simulink subsystem "VCM_main_Acc2"  (R2021b)
settings: Solver=VariableStepAuto  StartTime=0.0  StopTime=10.0  RelTol=1e-3
undefined symbols (not defined in the file): df, dr, g, gear_f, gear_r, Iwf, Iwr, l, lf, M, Rwf, Rwr
libraries: simulink x43, dspstat3 x2, dspswit3 x1
(part 1 of 3)
settings Model: Creator=tsuyoshi  LastModifiedBy=FEM

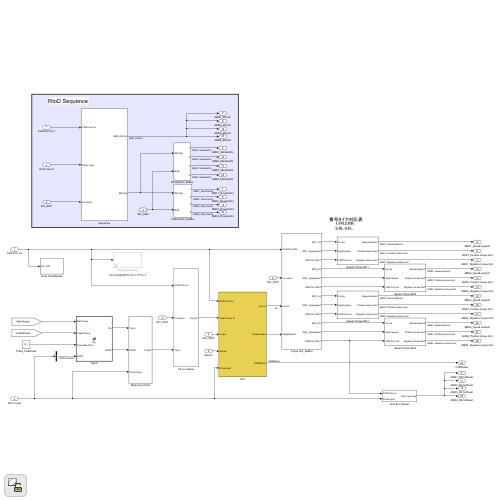
[thumbnail: Simulink's stored preview of the top-level diagram]
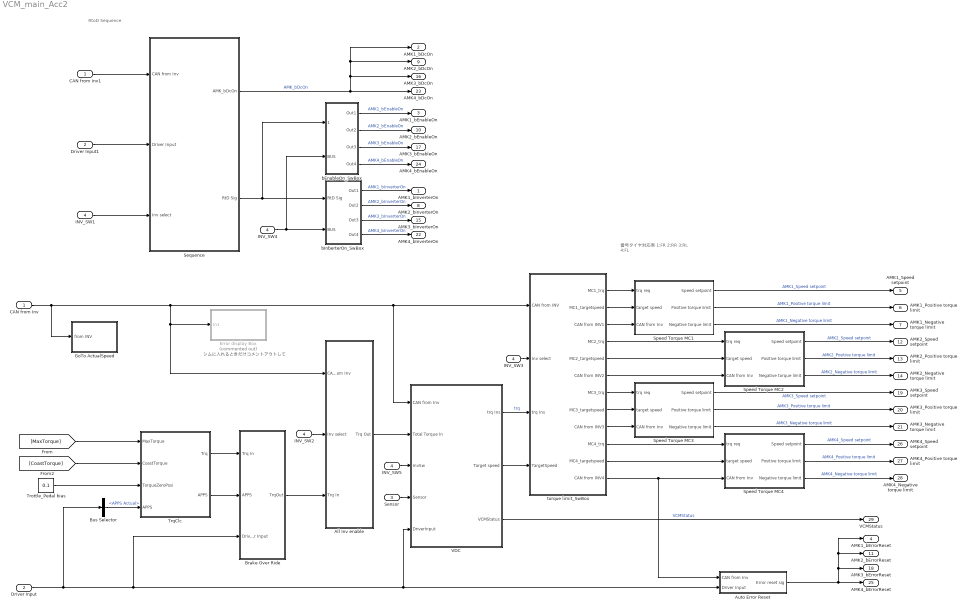
== system VCM_main_Acc2 ==
  note: シムに入れるときだけコメントアウトして
  note: RtoD Sequence
  note: 番号タイヤ対応表
      | 1:FR 2:RR
      | 3:RL 4:FL
  CAN from Inv : Inport
  Driver Input : Inport  Port=2
  Sensor : Inport  Port=3
  INV_SW1 : Inport  Port=4
  All Inv enable : Subsystem
  Auto Error Reset : Subsystem
  Brake Over Ride : Subsystem
  Bus Selector : BusSelector  OutputSignals=APPS Actual
  CAN from Inv1 : InportShadow
  Driver Input1 : InportShadow  Port=2
  Error display Box : Subsystem  Commented=on
  GoTo ActualSpeed : Subsystem
  INV_SW{2..5} (4 alike) : InportShadow  Port=4
  Sequence : Subsystem
  Speed Torque MC1 : Subsystem
  Speed Torque MC2 : Subsystem
  Speed Torque MC3 : Subsystem
  Speed Torque MC4 : Subsystem
  Trottle_Pedal bias : Constant  Value=0.1
  TrqClc : MATLAB Function  TreatAsAtomicUnit=on
  VDC : Subsystem
  bEnableOn_SwBox : Subsystem
  bInberterOn_SwBox : Subsystem
  torque limit_SwBox : Subsystem
  AMK1_bInverterOn : Outport  VectorParamsAs1DForOutWhenUnconnected=off
  AMK1_bDcOn : Outport  Port=2  VectorParamsAs1DForOutWhenUnconnected=off
  AMK1_bEnableOn : Outport  Port=3  VectorParamsAs1DForOutWhenUnconnected=off
  AMK1_bErrorReset : Outport  Port=4  VectorParamsAs1DForOutWhenUnconnected=off
  AMK1_Speed setpoint : Outport  Port=5  VectorParamsAs1DForOutWhenUnconnected=off
  AMK1_Positive torque limit : Outport  Port=6  VectorParamsAs1DForOutWhenUnconnected=off
  AMK1_Negative torque limit : Outport  Port=7  VectorParamsAs1DForOutWhenUnconnected=off
  AMK2_bInverterOn : Outport  Port=8  VectorParamsAs1DForOutWhenUnconnected=off
  AMK2_bDcOn : Outport  Port=9  VectorParamsAs1DForOutWhenUnconnected=off
  AMK2_bEnableOn : Outport  Port=10  VectorParamsAs1DForOutWhenUnconnected=off
  AMK2_bErrorReset : Outport  Port=11  VectorParamsAs1DForOutWhenUnconnected=off
  AMK2_Speed setpoint : Outport  Port=12  VectorParamsAs1DForOutWhenUnconnected=off
  AMK2_Positive torque limit : Outport  Port=13  VectorParamsAs1DForOutWhenUnconnected=off
  AMK2_Negative torque limit : Outport  Port=14  VectorParamsAs1DForOutWhenUnconnected=off
  AMK3_bInverterOn : Outport  Port=15  VectorParamsAs1DForOutWhenUnconnected=off
  AMK3_bDcOn : Outport  Port=16  VectorParamsAs1DForOutWhenUnconnected=off
  AMK3_bEnableOn : Outport  Port=17  VectorParamsAs1DForOutWhenUnconnected=off
  AMK3_bErrorReset : Outport  Port=18  VectorParamsAs1DForOutWhenUnconnected=off
  AMK3_Speed setpoint : Outport  Port=19  VectorParamsAs1DForOutWhenUnconnected=off
  AMK3_Positive torque limit : Outport  Port=20  VectorParamsAs1DForOutWhenUnconnected=off
  AMK3_Negative torque limit : Outport  Port=21  VectorParamsAs1DForOutWhenUnconnected=off
  AMK4_bInverterOn : Outport  Port=22  VectorParamsAs1DForOutWhenUnconnected=off
  AMK4_bDcOn : Outport  Port=23  VectorParamsAs1DForOutWhenUnconnected=off
  AMK4_bEnableOn : Outport  Port=24  VectorParamsAs1DForOutWhenUnconnected=off
  AMK4_bErrorReset : Outport  Port=25  VectorParamsAs1DForOutWhenUnconnected=off
  AMK4_Speed setpoint : Outport  Port=26  VectorParamsAs1DForOutWhenUnconnected=off
  AMK4_Positive torque limit : Outport  Port=27  VectorParamsAs1DForOutWhenUnconnected=off
  AMK4_Negative torque limit : Outport  Port=28  VectorParamsAs1DForOutWhenUnconnected=off
  VCMStatus : Outport  Port=29  VectorParamsAs1DForOutWhenUnconnected=off
  wires:
  Sequence/1(AMK_bDcOn) -> AMK4_bDcOn/1, AMK3_bDcOn/1, AMK2_bDcOn/1, AMK1_bDcOn/1  "AMK_bDcOn"
  Trottle_Pedal bias/1 -> TrqClc/3(TorqueZeroPosi)
  bInberterOn_SwBox/1(Out1) -> AMK1_bInverterOn/1  "AMK1_bInverterOn"
  bInberterOn_SwBox/2(Out2) -> AMK2_bInverterOn/1  "AMK2_bInverterOn"
  bInberterOn_SwBox/3(Out3) -> AMK3_bInverterOn/1  "AMK3_bInverterOn"
  bInberterOn_SwBox/4(Out4) -> AMK4_bInverterOn/1  "AMK4_bInverterOn"
  INV_SW1/1 -> Sequence/3(Inv select)
  bEnableOn_SwBox/1(Out1) -> AMK1_bEnableOn/1  "AMK1_bEnableOn"
  bEnableOn_SwBox/2(Out2) -> AMK2_bEnableOn/1  "AMK2_bEnableOn"
  bEnableOn_SwBox/3(Out3) -> AMK3_bEnableOn/1  "AMK3_bEnableOn"
  bEnableOn_SwBox/4(Out4) -> AMK4_bEnableOn/1  "AMK4_bEnableOn"
  Sequence/2(RtD Sig) -> bEnableOn_SwBox/1(RtD Sig), bInberterOn_SwBox/1(RtD Sig)
  VDC/1(trq Ins) -> torque limit_SwBox/3(trq Ins)  "trq"
  CAN from Inv/1 -> GoTo ActualSpeed/1(from INV), torque limit_SwBox/1(CAN from INV), VDC/1(CAN from Inv), All Inv enable/1(CAN from Inv), Error display Box/1(In1)
  TrqClc/1(Trq) -> Brake Over Ride/1(Trq In)
  Brake Over Ride/1(TrqOut) -> All Inv enable/3(Trq In)
  All Inv enable/1(Trq Out) -> VDC/2(Total Torque In)
  torque limit_SwBox/1(MC1_trq) -> Speed Torque MC1/1(trq req)
  Speed Torque MC1/1(Speed setpoint) -> AMK1_Speed setpoint/1  "AMK1_Speed setpoint"
  Speed Torque MC1/2(Positive torque limit) -> AMK1_Positive torque limit/1  "AMK1_Positive torque limit"
  Speed Torque MC1/3(Negative torque limit) -> AMK1_Negative torque limit/1  "AMK1_Negative torque limit"
  Speed Torque MC2/1(Speed setpoint) -> AMK2_Speed setpoint/1  "AMK2_Speed setpoint"
  Speed Torque MC2/2(Positive torque limit) -> AMK2_Positive torque limit/1  "AMK2_Positive torque limit"
  Speed Torque MC2/3(Negative torque limit) -> AMK2_Negative torque limit/1  "AMK2_Negative torque limit"
  torque limit_SwBox/4(MC2_trq) -> Speed Torque MC2/1(trq req)
  Speed Torque MC3/1(Speed setpoint) -> AMK3_Speed setpoint/1  "AMK3_Speed setpoint"
  Speed Torque MC3/2(Positive torque limit) -> AMK3_Positive torque limit/1  "AMK3_Positive torque limit"
  Speed Torque MC3/3(Negative torque limit) -> AMK3_Negative torque limit/1  "AMK3_Negative torque limit"
  Speed Torque MC4/1(Speed setpoint) -> AMK4_Speed setpoint/1  "AMK4_Speed setpoint"
  Speed Torque MC4/2(Positive torque limit) -> AMK4_Positive torque limit/1  "AMK4_Positive torque limit"
  Speed Torque MC4/3(Negative torque limit) -> AMK4_Negative torque limit/1  "AMK4_Negative torque limit"
  torque limit_SwBox/7(MC3_trq) -> Speed Torque MC3/1(trq req)
  torque limit_SwBox/10(MC4_trq) -> Speed Torque MC4/1(trq req)
  Auto Error Reset/1(Error reset sig) -> AMK4_bErrorReset/1, AMK3_bErrorReset/1, AMK1_bErrorReset/1, AMK2_bErrorReset/1
  Sensor/1 -> VDC/4(Sensor)
  torque limit_SwBox/2(MC1_targetspeed) -> Speed Torque MC1/2(target speed)
  torque limit_SwBox/8(MC3_targetspeed) -> Speed Torque MC3/2(target speed)
  torque limit_SwBox/5(MC2_targetspeed) -> Speed Torque MC2/2(target speed)
  torque limit_SwBox/11(MC4_targetspeed) -> Speed Torque MC4/2(target speed)
  VDC/3(VCMStatus) -> VCMStatus/1  "VCMStatus"
  VDC/2(Target speed) -> torque limit_SwBox/4(TargetSpeed)
  INV_SW2/1 -> All Inv enable/2(Inv select)
  INV_SW3/1 -> torque limit_SwBox/2(Inv select)
  INV_SW4/1 -> bInberterOn_SwBox/2(BUS), bEnableOn_SwBox/2(BUS)
  torque limit_SwBox/3(CAN from INV1) -> Speed Torque MC1/3(CAN from Inv)
  torque limit_SwBox/6(CAN from INV2) -> Speed Torque MC2/3(CAN from Inv)
  torque limit_SwBox/9(CAN from INV3) -> Speed Torque MC3/3(CAN from Inv)
  torque limit_SwBox/12(CAN from INV4) -> Auto Error Reset/1(CAN from Inv), Speed Torque MC4/3(CAN from Inv)
  [MaxTorque] -> TrqClc/1(MaxTorque)
  Driver Input1/1 -> Sequence/2(Driver Input)
  CAN from Inv1/1 -> Sequence/1(CAN from Inv)
  [CoastTorque] -> TrqClc/2(CoastTorque)
  Bus Selector/1 -> TrqClc/4("APPS ")  "<APPS Actual>"
  TrqClc/2(APPS) -> Brake Over Ride/2(APPS)
  INV_SW5/1 -> VDC/3(InvSw)
  Driver Input/1 -> Brake Over Ride/3(Driver Input), VDC/5(DriverInput), Auto Error Reset/2(Driver Input), Bus Selector/1

== system VCM_main_Acc2/All Inv enable ==
  note: インバータがQuitInverterOnになる前にトルク指令値を送ってはいけない
  CAN from Inv : Inport
  Inv select : Inport  Port=2
  Trq In : Inport  Port=3
  All Inv enable : Subsystem
  Constant : Constant  Value=0
  Switch : Switch  Criteria=u2 ~= 0
  Trq Out : Outport  VectorParamsAs1DForOutWhenUnconnected=off
  wires:
  CAN from Inv/1 -> All Inv enable/1(CAN from Inv)
  Inv select/1 -> All Inv enable/2(Inv select)
  Trq In/1 -> Switch/1
  Switch/1 -> Trq Out/1
  All Inv enable/1(Out1) -> Switch/2
  Constant/1 -> Switch/3

== system VCM_main_Acc2/Auto Error Reset ==
  note: AutoErrorResetにしたいときは
      | これを下につなげる
  CAN from Inv : Inport
  Driver Input : Inport  Port=2
  Bus Selector : BusSelector  OutputSignals=ErrorResetSW
  Bus Selector1 : BusSelector  OutputSignals=MC_11.MC1_bError,MC_21.MC2_bError,MC_31.MC3_bError,MC_41.MC4_bError
  Counter : dspswit3/Counter  Direction=Up  CountEvent=Rising edge  CounterSize=User defined  MaxCount=5  InitialCount=0  Output=Hit  HitValue=5  ResetInput=on  SamplesPerFrame=1  Ts=1  CntDtype=double  HitDtype=Logical
  Data Type Conversion : DataTypeConversion  OutMin=[0]  OutMax=[1]  OutDataTypeStr=double
  Delay : Delay  DelayLength=1  InitialCondition=0
  Logical Operator : Logic  Operator=OR  AllPortsSameDT=off  OutDataTypeStr=boolean
  Logical Operator1 : Logic  Operator=OR  Inputs=4  AllPortsSameDT=off  OutDataTypeStr=boolean
  Logical Operator2 : Logic  AllPortsSameDT=off  OutDataTypeStr=boolean
  Logical Operator3 : Logic  Operator=NOT  AllPortsSameDT=off  OutDataTypeStr=boolean
  Logical Operator4 : Logic  Operator=OR  AllPortsSameDT=off  OutDataTypeStr=boolean
  Pulse Generator : DiscretePulseGenerator  PulseType=Time based  Period=60  PulseWidth=5
  Terminator : Terminator
  Error reset sig : Outport  VectorParamsAs1DForOutWhenUnconnected=off
  wires:
  Logical Operator/1 -> Terminator/1
  Data Type Conversion/1 -> Error reset sig/1  "AMK_bErrorReset"
  Bus Selector1/4 -> Logical Operator1/4  "<MC4_bError>"
  Bus Selector1/3 -> Logical Operator1/3  "<MC3_bError>"
  Bus Selector1/1 -> Logical Operator1/1  "<MC1_bError>"
  Bus Selector1/2 -> Logical Operator1/2  "<MC2_bError>"
  Pulse Generator/1 -> Counter/2
  Delay/1 -> Logical Operator4/2
  Counter/1 -> Logical Operator4/1
  Logical Operator4/1 -> Delay/1, Logical Operator3/1
  Logical Operator2/1 -> Logical Operator/1
  Logical Operator3/1 -> Logical Operator2/2
  Logical Operator1/1 -> Counter/1, Logical Operator2/1
  CAN from Inv/1 -> Bus Selector1/1
  Bus Selector/1 -> Logical Operator/2, Data Type Conversion/1  "<ErrorResetSW>"
  Driver Input/1 -> Bus Selector/1

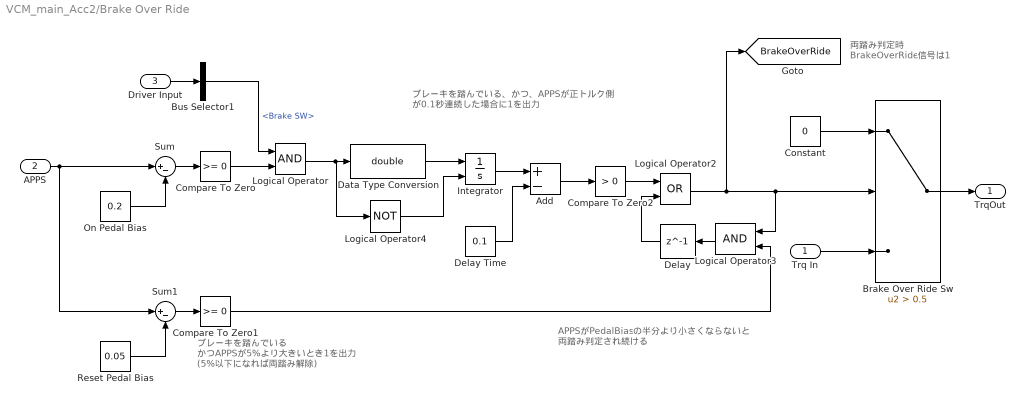
== system VCM_main_Acc2/Brake Over Ride ==
  note: APPSがPedalBiasの半分より小さくならないと
      | 両踏み判定され続ける
  note: ブレーキを踏んでいる
      | かつAPPSが5%より大きいとき1を出力
      | (5%以下になれば両踏み解除)
  note: 両踏み判定時
      | BrakeOverRide信号は1
  note: ブレーキを踏んでいる、かつ、APPSが正トルク側
      | が0.1秒連続した場合に1を出力
  Trq In : Inport
  APPS : Inport  Port=2
  Driver Input : Inport  Port=3
  Add : Sum  Inputs=+-
  Brake Over Ride Sw : Switch  Criteria=u2 > Threshold  Threshold=0.5
  Bus Selector1 : BusSelector  OutputSignals=Brake SW
  Compare To Zero : simulink/Logic and Bit Operations/Compare To Zero  relop=>=  OutDataTypeStr=boolean
  Compare To Zero1 : simulink/Logic and Bit Operations/Compare To Zero  relop=>=  OutDataTypeStr=boolean
  Compare To Zero2 : simulink/Logic and Bit Operations/Compare To Zero  relop=>  OutDataTypeStr=boolean
  Constant : Constant  Value=0
  Data Type Conversion : DataTypeConversion  OutDataTypeStr=double
  Delay : Delay  DelayLength=1  InitialCondition=0
  Delay Time : Constant  Value=0.1
  Integrator : Integrator  ExternalReset=rising
  Logical Operator : Logic  AllPortsSameDT=off  OutDataTypeStr=boolean
  Logical Operator2 : Logic  Operator=OR  AllPortsSameDT=off  OutDataTypeStr=boolean
  Logical Operator3 : Logic  AllPortsSameDT=off  OutDataTypeStr=boolean
  Logical Operator4 : Logic  Operator=NOT  AllPortsSameDT=off  OutDataTypeStr=boolean
  On Pedal Bias : Constant  Value=0.2
  Reset Pedal Bias : Constant  Value=0.05
  Sum : Sum  Inputs=|+-
  Sum1 : Sum  Inputs=|+-
  TrqOut : Outport  VectorParamsAs1DForOutWhenUnconnected=off
  tag scope: BrakeOverRide=global
  wires:
  Constant/1 -> Brake Over Ride Sw/1
  Brake Over Ride Sw/1 -> TrqOut/1
  Delay Time/1 -> Add/2
  Logical Operator/1 -> Data Type Conversion/1, Logical Operator4/1
  Integrator/1 -> Add/1
  Reset Pedal Bias/1 -> Sum1/2
  Sum/1 -> Compare To Zero/1
  Driver Input/1 -> Bus Selector1/1
  Logical Operator4/1 -> Integrator/2
  Logical Operator3/1 -> Delay/1
  Trq In/1 -> Brake Over Ride Sw/3
  Bus Selector1/1 -> Logical Operator/1  "<Brake SW>"
  APPS/1 -> Sum1/1, Sum/1
  Delay/1 -> Logical Operator2/2
  Data Type Conversion/1 -> Integrator/1
  Sum1/1 -> Compare To Zero1/1
  Compare To Zero2/1 -> Logical Operator2/1
  Compare To Zero/1 -> Logical Operator/2
  On Pedal Bias/1 -> Sum/2
  Logical Operator2/1 -> [BrakeOverRide], Logical Operator3/1, Brake Over Ride Sw/2
  Compare To Zero1/1 -> Logical Operator3/2
  Add/1 -> Compare To Zero2/1

== system VCM_main_Acc2/Error display Box ==
  note: 過去のエラーメッセージを見れるようにするためにある
  In1 : Inport
  All system ready : Logic  Inputs=4  AllPortsSameDT=off  OutDataTypeStr=boolean
  Bus Selector : BusSelector  OutputSignals=MC_11.MC1_bSystemReady,MC_21.MC2_bSystemReady,MC_31.MC3_bSystemReady,MC_41.MC4_bSystemReady
  Display : Display
  Error Info : Subsystem
  Error Info Display{,1..3} (4 alike) : Display
  Error Info1 : Subsystem
  Error Info2 : Subsystem
  Error Info3 : Subsystem
  wires:
  All system ready/1 -> Display/1
  Bus Selector/4 -> All system ready/4  "<MC4_bSystemReady>"
  Bus Selector/3 -> All system ready/3  "<MC3_bSystemReady>"
  Bus Selector/2 -> All system ready/2  "<MC2_bSystemReady>"
  Bus Selector/1 -> All system ready/1  "<MC1_bSystemReady>"
  Error Info/2(Out2) -> Error Info3/2(In2), Error Info2/2(In2), Error Info1/2(In2)
  Error Info3/1(Out1) -> Error Info Display3/1
  Error Info2/1(Out1) -> Error Info Display2/1
  Error Info1/1(Out1) -> Error Info Display1/1
  In1/1 -> Error Info/1(In1), Error Info1/1(In1), Error Info2/1(In1), Error Info3/1(In1), Bus Selector/1
  Error Info/1(Out1) -> Error Info Display/1

== system VCM_main_Acc2/GoTo ActualSpeed ==
  note: 番号タイヤ対応表
      | 1:FR 2:RR
      | 3:RL 4:FL
  from INV : Inport
  Bus Selector : BusSelector  OutputSignals=MC_11.MC1_Actual speed value in 1/rpm,MC_21.MC2_Actual speed value in 1/rpm,MC_31.MC3_Actual speed value in 1/rpm,MC_41.MC4_Actual speed value in 1/rpm
  tag scope: FL_ActualSpeed=global, FR_ActualSpeed=global, RL_ActualSpeed=global, RR_ActualSpeed=global
  wires:
  Bus Selector/4 -> [FL_ActualSpeed]  "<MC4_Actual speed value in 1/rpm>"
  Bus Selector/3 -> [RL_ActualSpeed]  "<MC3_Actual speed value in 1/rpm>"
  Bus Selector/2 -> [RR_ActualSpeed]  "<MC2_Actual speed value in 1/rpm>"
  Bus Selector/1 -> [FR_ActualSpeed]  "<MC1_Actual speed value in 1/rpm>"
  from INV/1 -> Bus Selector/1

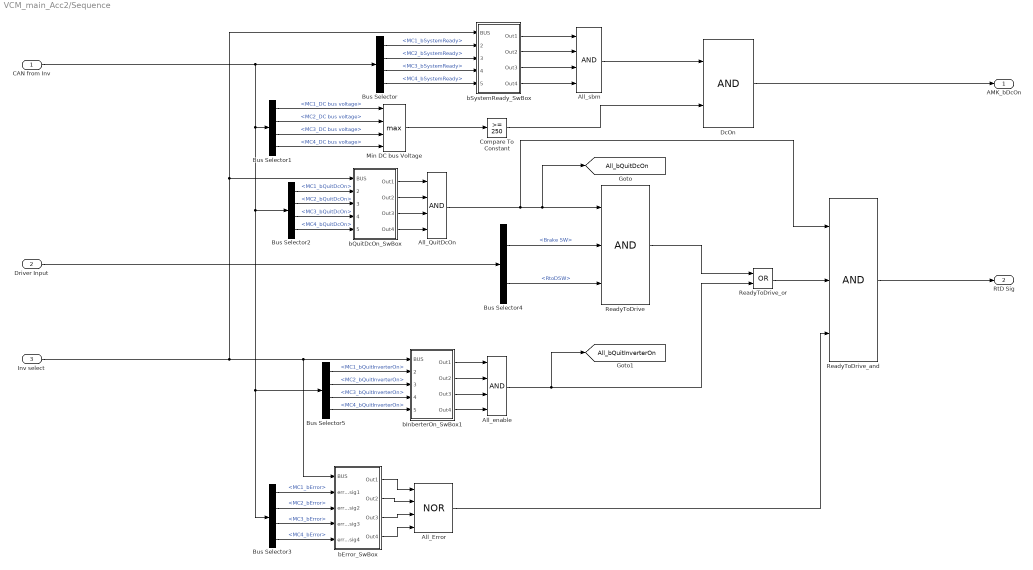
== system VCM_main_Acc2/Sequence ==
  CAN from Inv : Inport
  Driver Input : Inport  Port=2
  Inv select : Inport  Port=3
  All_Error : Logic  Operator=NOR  Inputs=4  AllPortsSameDT=off  OutDataTypeStr=boolean
  All_QuitDcOn : Logic  Inputs=4  AllPortsSameDT=off  OutDataTypeStr=boolean
  All_enable : Logic  Inputs=4  AllPortsSameDT=off  OutDataTypeStr=boolean
  All_sbm : Logic  Inputs=4  AllPortsSameDT=off  OutDataTypeStr=boolean
  Bus Selector : BusSelector  OutputSignals=MC_11.MC1_bSystemReady,MC_21.MC2_bSystemReady,MC_31.MC3_bSystemReady,MC_41.MC4_bSystemReady
  Bus Selector1 : BusSelector  OutputSignals=MC_11.MC1_DC bus voltage,MC_21.MC2_DC bus voltage,MC_31.MC3_DC bus voltage,MC_41.MC4_DC bus voltage
  Bus Selector2 : BusSelector  OutputSignals=MC_11.MC1_bQuitDcOn,MC_21.MC2_bQuitDcOn,MC_31.MC3_bQuitDcOn,MC_41.MC4_bQuitDcOn
  Bus Selector3 : BusSelector  OutputSignals=MC_11.MC1_bError,MC_21.MC2_bError,MC_31.MC3_bError,MC_41.MC4_bError
  Bus Selector4 : BusSelector  OutputSignals=Brake SW,RtoDSW
  Bus Selector5 : BusSelector  OutputSignals=MC_11.MC1_bQuitInverterOn,MC_21.MC2_bQuitInverterOn,MC_31.MC3_bQuitInverterOn,MC_41.MC4_bQuitInverterOn
  Compare To Constant : simulink/Logic and Bit Operations/Compare To Constant  relop=>=  const=250  OutDataTypeStr=boolean
  DcOn : Logic  AllPortsSameDT=off  OutDataTypeStr=boolean
  Min DC bus Voltage : MinMax  Function=max  Inputs=4
  ReadyToDrive : Logic  Inputs=3  AllPortsSameDT=off  OutDataTypeStr=boolean
  ReadyToDrive_and : Logic  Inputs=3  AllPortsSameDT=off  OutDataTypeStr=boolean
  ReadyToDrive_or : Logic  Operator=OR  AllPortsSameDT=off  OutDataTypeStr=boolean
  bError_SwBox : Subsystem
  bInberterOn_SwBox1 : Subsystem
  bQuitDcOn_SwBox : Subsystem
  bSystemReady_SwBox : Subsystem
  AMK_bDcOn : Outport  VectorParamsAs1DForOutWhenUnconnected=off
  RtD Sig : Outport  Port=2  VectorParamsAs1DForOutWhenUnconnected=off
  tag scope: All_bQuitDcOn=global, All_bQuitInverterOn=global
  wires:
  Inv select/1 -> bError_SwBox/1(BUS), bInberterOn_SwBox1/1(BUS), bQuitDcOn_SwBox/1(BUS), bSystemReady_SwBox/1(BUS)
  bSystemReady_SwBox/4(Out4) -> All_sbm/4
  bSystemReady_SwBox/3(Out3) -> All_sbm/3
  bSystemReady_SwBox/2(Out2) -> All_sbm/2
  bSystemReady_SwBox/1(Out1) -> All_sbm/1
  Bus Selector/4 -> bSystemReady_SwBox/5(error sig4)  "<MC4_bSystemReady>"
  Bus Selector/3 -> bSystemReady_SwBox/4(error sig3)  "<MC3_bSystemReady>"
  Bus Selector/2 -> bSystemReady_SwBox/3(error sig2)  "<MC2_bSystemReady>"
  Bus Selector/1 -> bSystemReady_SwBox/2(error sig1)  "<MC1_bSystemReady>"
  bQuitDcOn_SwBox/4(Out4) -> All_QuitDcOn/4
  bQuitDcOn_SwBox/3(Out3) -> All_QuitDcOn/3
  bQuitDcOn_SwBox/2(Out2) -> All_QuitDcOn/2
  bQuitDcOn_SwBox/1(Out1) -> All_QuitDcOn/1
  Bus Selector2/4 -> bQuitDcOn_SwBox/5(error sig4)  "<MC4_bQuitDcOn>"
  Bus Selector2/3 -> bQuitDcOn_SwBox/4(error sig3)  "<MC3_bQuitDcOn>"
  Bus Selector2/2 -> bQuitDcOn_SwBox/3(error sig2)  "<MC2_bQuitDcOn>"
  Bus Selector2/1 -> bQuitDcOn_SwBox/2(error sig1)  "<MC1_bQuitDcOn>"
  Bus Selector5/4 -> bInberterOn_SwBox1/5(error sig4)  "<MC4_bQuitInverterOn>"
  Bus Selector5/3 -> bInberterOn_SwBox1/4(error sig3)  "<MC3_bQuitInverterOn>"
  Bus Selector5/1 -> bInberterOn_SwBox1/2(error sig1)  "<MC1_bQuitInverterOn>"
  Bus Selector5/2 -> bInberterOn_SwBox1/3(error sig2)  "<MC2_bQuitInverterOn>"
  bInberterOn_SwBox1/4(Out4) -> All_enable/4
  bInberterOn_SwBox1/3(Out3) -> All_enable/3
  bInberterOn_SwBox1/2(Out2) -> All_enable/2
  bInberterOn_SwBox1/1(Out1) -> All_enable/1
  All_enable/1 -> ReadyToDrive_or/2, [All_bQuitInverterOn]
  ReadyToDrive/1 -> ReadyToDrive_or/1
  ReadyToDrive_or/1 -> ReadyToDrive_and/2
  bError_SwBox/4(Out4) -> All_Error/4
  bError_SwBox/3(Out3) -> All_Error/3
  bError_SwBox/2(Out2) -> All_Error/2
  bError_SwBox/1(Out1) -> All_Error/1
  Bus Selector3/4 -> bError_SwBox/5(error sig4)  "<MC4_bError>"
  Bus Selector3/3 -> bError_SwBox/4(error sig3)  "<MC3_bError>"
  Bus Selector3/1 -> bError_SwBox/2(error sig1)  "<MC1_bError>"
  Bus Selector3/2 -> bError_SwBox/3(error sig2)  "<MC2_bError>"
  Bus Selector4/2 -> ReadyToDrive/3  "<RtoDSW>"
  Bus Selector4/1 -> ReadyToDrive/2  "<Brake SW>"
  Driver Input/1 -> Bus Selector4/1
  Bus Selector1/4 -> Min DC bus Voltage/4  "<MC4_DC bus voltage>"
  Bus Selector1/3 -> Min DC bus Voltage/3  "<MC3_DC bus voltage>"
  Bus Selector1/2 -> Min DC bus Voltage/2  "<MC2_DC bus voltage>"
  Bus Selector1/1 -> Min DC bus Voltage/1  "<MC1_DC bus voltage>"
  CAN from Inv/1 -> Bus Selector1/1, Bus Selector2/1, Bus Selector5/1, Bus Selector3/1, Bus Selector/1
  Min DC bus Voltage/1 -> Compare To Constant/1
  All_Error/1 -> ReadyToDrive_and/3
  Compare To Constant/1 -> DcOn/2
  ReadyToDrive_and/1 -> RtD Sig/1
  All_QuitDcOn/1 -> ReadyToDrive_and/1, [All_bQuitDcOn], ReadyToDrive/1
  DcOn/1 -> AMK_bDcOn/1
  All_sbm/1 -> DcOn/1

== system VCM_main_Acc2/Speed Torque MC1 ==
  note: 0.1%Mnに変換し、整数化
      | 0.1%MNはモーターの定格(9.8Nm)の
      | 何倍かを表す数に1000をかけたもの
  trq req : Inport
  target speed : Inport  Port=2
  CAN from Inv : Inport  Port=3
  Bus Selector : BusSelector  OutputSignals=MC_11.MC1_Actual speed value in 1/rpm
  Gain2 : Gain  Gain=1000/9.8
  Gain6 : Gain  Gain=1000/9.8
  Power limit Negative : Subsystem
  Power limit Positive : Subsystem
  Quantizer1 : Quantizer  QuantizationInterval=1
  Quantizer2 : Quantizer  QuantizationInterval=1
  Subsystem : Subsystem
  TargetVelocity : Subsystem
  Torque delay N : Subsystem
  Torque delay P : Subsystem
  Speed setpoint : Outport  VectorParamsAs1DForOutWhenUnconnected=off
  Positive torque limit : Outport  Port=2  VectorParamsAs1DForOutWhenUnconnected=off
  Negative torque limit : Outport  Port=3  VectorParamsAs1DForOutWhenUnconnected=off
  wires:
  Subsystem/1(Positive torque limit1) -> Positive torque limit/1  "Positive torque limit"
  Torque delay P/1(Out1) -> Subsystem/1(Positive torque limit)
  Torque delay N/1(Out1) -> Negative torque limit/1  "Negative torque limit"
  Bus Selector/1 -> Power limit Positive/2(Speed), Power limit Negative/1(Speed)  "<MC1_Actual speed value in 1/rpm>"
  CAN from Inv/1 -> Bus Selector/1
  target speed/1 -> TargetVelocity/2(target speed)
  Power limit Positive/1(Out1) -> Gain2/1
  trq req/1 -> Power limit Negative/2(Trq), Power limit Positive/1(Trq)
  Gain6/1 -> Quantizer2/1
  Power limit Negative/1(Out1) -> Gain6/1
  Gain2/1 -> Quantizer1/1
  TargetVelocity/1(SpeedSetpoint) -> Speed setpoint/1  "Speed setpoint"
  Quantizer2/1 -> Torque delay N/1(In1)
  Quantizer1/1 -> Torque delay P/1(In1), TargetVelocity/1(trq)

== system VCM_main_Acc2/Speed Torque MC2 ==
  note: 0.1%Mnに変換し、整数化
      | 0.1%MNはモーターの定格(9.8Nm)の
      | 何倍かを表す数に1000をかけたもの
  trq req : Inport
  target speed : Inport  Port=2
  CAN from Inv : Inport  Port=3
  Bus Selector : BusSelector  OutputSignals=MC_21.MC2_Actual speed value in 1/rpm
  Gain2 : Gain  Gain=1000/9.8
  Gain6 : Gain  Gain=1000/9.8
  Power limit Negative : Subsystem
  Power limit Positive : Subsystem
  Quantizer1 : Quantizer  QuantizationInterval=1
  Quantizer2 : Quantizer  QuantizationInterval=1
  Subsystem : Subsystem
  TargetVelocity : Subsystem
  Torque delay N : Subsystem
  Torque delay P : Subsystem
  Speed setpoint : Outport  VectorParamsAs1DForOutWhenUnconnected=off
  Positive torque limit : Outport  Port=2  VectorParamsAs1DForOutWhenUnconnected=off
  Negative torque limit : Outport  Port=3  VectorParamsAs1DForOutWhenUnconnected=off
  wires:
  Quantizer1/1 -> TargetVelocity/1(trq), Torque delay P/1(In1)
  Quantizer2/1 -> Torque delay N/1(In1)
  TargetVelocity/1(SpeedSetpoint) -> Speed setpoint/1  "Speed setpoint"
  Gain2/1 -> Quantizer1/1
  Power limit Negative/1(Out1) -> Gain6/1
  Gain6/1 -> Quantizer2/1
  trq req/1 -> Power limit Positive/1(Trq), Power limit Negative/2(Trq)
  Power limit Positive/1(Out1) -> Gain2/1
  target speed/1 -> TargetVelocity/2(target speed)
  CAN from Inv/1 -> Bus Selector/1
  Bus Selector/1 -> Power limit Negative/1(Speed), Power limit Positive/2(Speed)  "<MC2_Actual speed value in 1/rpm>"
  Torque delay N/1(Out1) -> Negative torque limit/1  "Negative torque limit"
  Torque delay P/1(Out1) -> Subsystem/1(Positive torque limit)
  Subsystem/1(Positive torque limit1) -> Positive torque limit/1  "Positive torque limit"

== system VCM_main_Acc2/Speed Torque MC3 ==
  note: 0.1%Mnに変換し、整数化
      | 0.1%MNはモーターの定格(9.8Nm)の
      | 何倍かを表す数に1000をかけたもの
  trq req : Inport
  target speed : Inport  Port=2
  CAN from Inv : Inport  Port=3
  Bus Selector : BusSelector  OutputSignals=MC_31.MC3_Actual speed value in 1/rpm
  Gain2 : Gain  Gain=1000/9.8
  Gain6 : Gain  Gain=1000/9.8
  Power limit Negative : Subsystem
  Power limit Positive : Subsystem
  Quantizer1 : Quantizer  QuantizationInterval=1
  Quantizer2 : Quantizer  QuantizationInterval=1
  Subsystem : Subsystem
  TargetVelocity : Subsystem
  Torque delay N : Subsystem
  Torque delay P : Subsystem
  Speed setpoint : Outport  VectorParamsAs1DForOutWhenUnconnected=off
  Positive torque limit : Outport  Port=2  VectorParamsAs1DForOutWhenUnconnected=off
  Negative torque limit : Outport  Port=3  VectorParamsAs1DForOutWhenUnconnected=off
  wires:
  Subsystem/1(Positive torque limit1) -> Positive torque limit/1  "Positive torque limit"
  Torque delay P/1(Out1) -> Subsystem/1(Positive torque limit)
  Torque delay N/1(Out1) -> Negative torque limit/1  "Negative torque limit"
  Bus Selector/1 -> Power limit Positive/2(Speed), Power limit Negative/1(Speed)  "<MC3_Actual speed value in 1/rpm>"
  CAN from Inv/1 -> Bus Selector/1
  target speed/1 -> TargetVelocity/2(target speed)
  Power limit Positive/1(Out1) -> Gain2/1
  trq req/1 -> Power limit Negative/2(Trq), Power limit Positive/1(Trq)
  Gain6/1 -> Quantizer2/1
  Power limit Negative/1(Out1) -> Gain6/1
  Gain2/1 -> Quantizer1/1
  TargetVelocity/1(SpeedSetpoint) -> Speed setpoint/1  "Speed setpoint"
  Quantizer2/1 -> Torque delay N/1(In1)
  Quantizer1/1 -> Torque delay P/1(In1), TargetVelocity/1(trq)

== system VCM_main_Acc2/Speed Torque MC4 ==
  note: 0.1%Mnに変換し、整数化
      | 0.1%MNはモーターの定格(9.8Nm)の
      | 何倍かを表す数に1000をかけたもの
  trq req : Inport
  target speed : Inport  Port=2
  CAN from Inv : Inport  Port=3
  Bus Selector : BusSelector  OutputSignals=MC_41.MC4_Actual speed value in 1/rpm
  Gain2 : Gain  Gain=1000/9.8
  Gain6 : Gain  Gain=1000/9.8
  Power limit Negative : Subsystem
  Power limit Positive : Subsystem
  Quantizer1 : Quantizer  QuantizationInterval=1
  Quantizer2 : Quantizer  QuantizationInterval=1
  Subsystem : Subsystem
  TargetVelocity : Subsystem
  Torque delay N : Subsystem
  Torque delay P : Subsystem
  Speed setpoint : Outport  VectorParamsAs1DForOutWhenUnconnected=off
  Positive torque limit : Outport  Port=2  VectorParamsAs1DForOutWhenUnconnected=off
  Negative torque limit : Outport  Port=3  VectorParamsAs1DForOutWhenUnconnected=off
  wires:
  Quantizer1/1 -> TargetVelocity/1(trq), Torque delay P/1(In1)
  Quantizer2/1 -> Torque delay N/1(In1)
  TargetVelocity/1(SpeedSetpoint) -> Speed setpoint/1  "Speed setpoint"
  Gain2/1 -> Quantizer1/1
  Power limit Negative/1(Out1) -> Gain6/1
  Gain6/1 -> Quantizer2/1
  trq req/1 -> Power limit Positive/1(Trq), Power limit Negative/2(Trq)
  Power limit Positive/1(Out1) -> Gain2/1
  target speed/1 -> TargetVelocity/2(target speed)
  CAN from Inv/1 -> Bus Selector/1
  Bus Selector/1 -> Power limit Negative/1(Speed), Power limit Positive/2(Speed)  "<MC4_Actual speed value in 1/rpm>"
  Torque delay N/1(Out1) -> Negative torque limit/1  "Negative torque limit"
  Torque delay P/1(Out1) -> Subsystem/1(Positive torque limit)
  Subsystem/1(Positive torque limit1) -> Positive torque limit/1  "Positive torque limit"

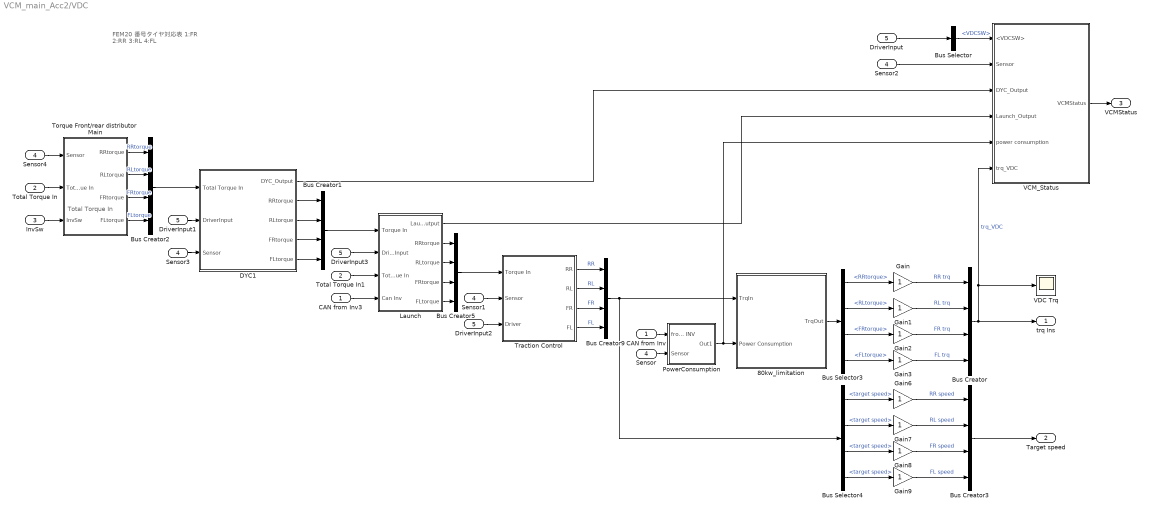
== system VCM_main_Acc2/VDC ==
  note: FEM20
      | 番号タイヤ対応表
      | 1:FR 2:RR
      | 3:RL 4:FL
  note: Total Torque In
  CAN from Inv : Inport
  Total Torque In : Inport  Port=2
  InvSw : Inport  Port=3
  Sensor : Inport  Port=4
  DriverInput : Inport  Port=5
  80kw_limitation : Subsystem
  Bus Creator{,1..3,5,9} (6 alike) : BusCreator  Inputs=4
  Bus Selector : BusSelector  OutputSignals=VDCSW
  Bus Selector3 : BusSelector  OutputSignals=RRtorque,RLtorque,FRtorque,FLtorque
  Bus Selector4 : BusSelector  OutputSignals=RR.target speed,RL.target speed,FR.target speed,FL.target speed
  CAN from Inv3 : InportShadow
  DYC1 : Subsystem
  DriverInput1 : InportShadow  Port=5
  DriverInput2 : InportShadow  Port=5
  DriverInput3 : InportShadow  Port=5
  Gain{,1..3,6..9} (8 alike) : Gain
  Launch : Subsystem
  PowerConsumption : Subsystem
  Sensor{1..4} (4 alike) : InportShadow  Port=4
  Torque Front/rear distributor Main : Subsystem
  Total Torque In1 : InportShadow  Port=2
  Traction Control : Subsystem
  VCM_Status : Subsystem
  VDC Trq : Scope
  trq Ins : Outport  VectorParamsAs1DForOutWhenUnconnected=off
  Target speed : Outport  Port=2  VectorParamsAs1DForOutWhenUnconnected=off
  VCMStatus : Outport  Port=3  VectorParamsAs1DForOutWhenUnconnected=off
  wires:
  InvSw/1 -> Torque Front/rear distributor Main/3(InvSw)
  DriverInput2/1 -> Traction Control/3(Driver)
  Launch/2(RRtorque) -> Bus Creator5/1
  Launch/5(FLtorque) -> Bus Creator5/4
  Launch/4(FRtorque) -> Bus Creator5/3
  Launch/3(RLtorque) -> Bus Creator5/2
  Bus Creator5/1 -> Traction Control/1(Torque In)
  Launch/1(Launch_Output) -> VCM_Status/4(Launch_Output)
  Total Torque In1/1 -> Launch/3(Total Torque In)
  CAN from Inv3/1 -> Launch/4(Can Inv)
  DriverInput3/1 -> Launch/2(DriverInput)
  Torque Front/rear distributor Main/4(FLtorque) -> Bus Creator2/4  "FLtorque"
  Torque Front/rear distributor Main/3(FRtorque) -> Bus Creator2/3  "FRtorque"
  Torque Front/rear distributor Main/2(RLtorque) -> Bus Creator2/2  "RLtorque"
  Torque Front/rear distributor Main/1(RRtorque) -> Bus Creator2/1  "RRtorque"
  Total Torque In/1 -> Torque Front/rear distributor Main/2(Total Torque In)
  Sensor4/1 -> Torque Front/rear distributor Main/1(Sensor)
  Bus Creator2/1 -> DYC1/1(Total Torque In)
  DYC1/1(DYC_Output) -> VCM_Status/3(DYC_Output)
  DYC1/5(FLtorque) -> Bus Creator1/4
  DYC1/4(FRtorque) -> Bus Creator1/3
  DYC1/3(RLtorque) -> Bus Creator1/2
  DYC1/2(RRtorque) -> Bus Creator1/1
  Sensor3/1 -> DYC1/3(Sensor)
  DriverInput1/1 -> DYC1/2(DriverInput)
  Sensor2/1 -> VCM_Status/2(Sensor)
  Bus Creator1/1 -> Launch/1(Torque In)
  Sensor1/1 -> Traction Control/2(Sensor)
  Traction Control/4(FL) -> Bus Creator9/4  "FL"
  Traction Control/3(FR) -> Bus Creator9/3  "FR"
  Traction Control/2(RL) -> Bus Creator9/2  "RL"
  Traction Control/1(RR) -> Bus Creator9/1  "RR"
  Bus Selector/1 -> VCM_Status/1(<VDCSW>)  "<VDCSW>"
  Sensor/1 -> PowerConsumption/2(Sensor)
  Bus Creator9/1 -> Bus Selector4/1, 80kw_limitation/1(TrqIn)
  PowerConsumption/1(Out1) -> 80kw_limitation/2(Power Consumption), VCM_Status/5(power consumption)
  CAN from Inv/1 -> PowerConsumption/1(from INV)
  VCM_Status/1(VCMStatus) -> VCMStatus/1
  DriverInput/1 -> Bus Selector/1
  Gain9/1 -> Bus Creator3/4  "FL speed"
  Gain8/1 -> Bus Creator3/3  "FR speed"
  Gain7/1 -> Bus Creator3/2  "RL speed"
  Gain6/1 -> Bus Creator3/1  "RR speed"
  Bus Creator3/1 -> Target speed/1
  Bus Selector4/4 -> Gain9/1  "<target speed>"
  Bus Selector4/3 -> Gain8/1  "<target speed>"
  Bus Selector4/2 -> Gain7/1  "<target speed>"
  Bus Selector4/1 -> Gain6/1  "<target speed>"
  Bus Selector3/4 -> Gain3/1  "<FLtorque>"
  Bus Selector3/3 -> Gain2/1  "<FRtorque>"
  Bus Selector3/2 -> Gain1/1  "<RLtorque>"
  Bus Selector3/1 -> Gain/1  "<RRtorque>"
  80kw_limitation/1(TrqOut) -> Bus Selector3/1
  Gain3/1 -> Bus Creator/4  "FL trq"
  Gain2/1 -> Bus Creator/3  "FR trq"
  Gain1/1 -> Bus Creator/2  "RL trq"
  Gain/1 -> Bus Creator/1  "RR trq"
  Bus Creator/1 -> VCM_Status/6(trq_VDC), VDC Trq/1, trq Ins/1  "trq_VDC"

== system VCM_main_Acc2/bEnableOn_SwBox ==
  RtD Sig : Inport
  BUS : Inport  Port=2
  Bus Selector2 : BusSelector  OutputSignals=MC1_sw,MC2_sw,MC3_sw,MC4_sw
  Constant : Constant  Value=0
  Switch{1..4} (4 alike) : Switch  Criteria=u2 > Threshold
  Out1 : Outport  VectorParamsAs1DForOutWhenUnconnected=off
  Out2 : Outport  Port=2  VectorParamsAs1DForOutWhenUnconnected=off
  Out3 : Outport  Port=3  VectorParamsAs1DForOutWhenUnconnected=off
  Out4 : Outport  Port=4  VectorParamsAs1DForOutWhenUnconnected=off
  wires:
  BUS/1 -> Bus Selector2/1
  Bus Selector2/4 -> Switch4/2  "<MC4_sw>"
  Bus Selector2/3 -> Switch3/2  "<MC3_sw>"
  Bus Selector2/1 -> Switch1/2  "<MC1_sw>"
  Bus Selector2/2 -> Switch2/2  "<MC2_sw>"
  Switch3/1 -> Out3/1
  Switch2/1 -> Out2/1
  RtD Sig/1 -> Switch1/1, Switch3/1, Switch4/1, Switch2/1
  Switch1/1 -> Out1/1
  Switch4/1 -> Out4/1
  Constant/1 -> Switch1/3, Switch2/3, Switch3/3, Switch4/3

== system VCM_main_Acc2/bInberterOn_SwBox ==
  RtD Sig : Inport
  BUS : Inport  Port=2
  Bus Selector2 : BusSelector  OutputSignals=MC1_sw,MC2_sw,MC3_sw,MC4_sw
  Constant : Constant  Value=0
  Switch{1..4} (4 alike) : Switch  Criteria=u2 > Threshold
  Out1 : Outport  VectorParamsAs1DForOutWhenUnconnected=off
  Out2 : Outport  Port=2  VectorParamsAs1DForOutWhenUnconnected=off
  Out3 : Outport  Port=3  VectorParamsAs1DForOutWhenUnconnected=off
  Out4 : Outport  Port=4  VectorParamsAs1DForOutWhenUnconnected=off
  wires:
  BUS/1 -> Bus Selector2/1
  Bus Selector2/4 -> Switch4/2  "<MC4_sw>"
  Bus Selector2/3 -> Switch3/2  "<MC3_sw>"
  Bus Selector2/1 -> Switch1/2  "<MC1_sw>"
  Bus Selector2/2 -> Switch2/2  "<MC2_sw>"
  Switch3/1 -> Out3/1
  Switch2/1 -> Out2/1
  RtD Sig/1 -> Switch1/1, Switch4/1, Switch3/1, Switch2/1
  Switch1/1 -> Out1/1
  Switch4/1 -> Out4/1
  Constant/1 -> Switch1/3, Switch2/3, Switch3/3, Switch4/3

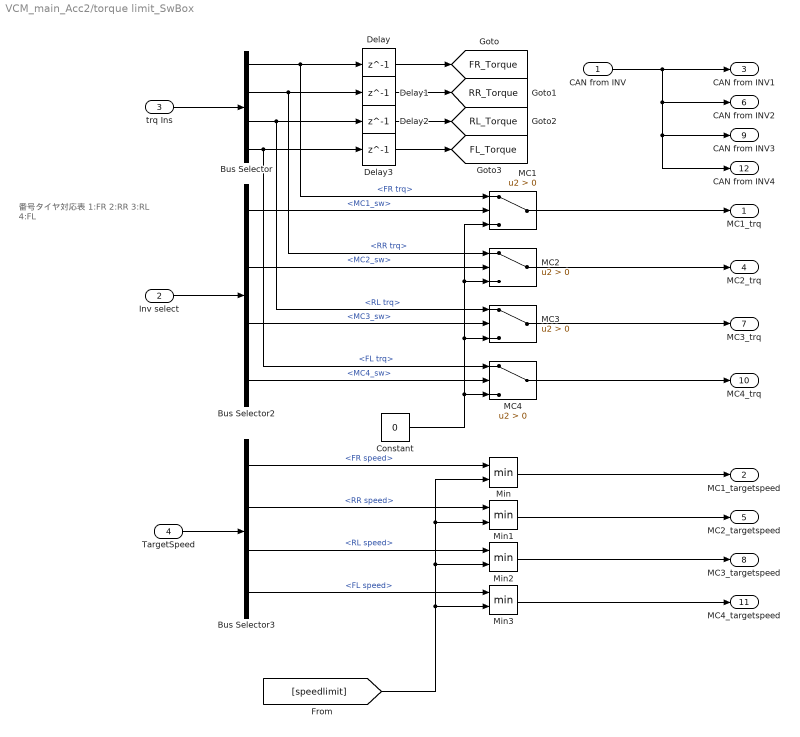
== system VCM_main_Acc2/torque limit_SwBox ==
  note: 番号タイヤ対応表
      | 1:FR 2:RR
      | 3:RL 4:FL
  CAN from INV : Inport
  Inv select : Inport  Port=2
  trq Ins : Inport  Port=3
  TargetSpeed : Inport  Port=4
  Bus Selector : BusSelector  OutputSignals=FR trq,RR trq,RL trq,FL trq
  Bus Selector2 : BusSelector  OutputSignals=MC1_sw,MC2_sw,MC3_sw,MC4_sw
  Bus Selector3 : BusSelector  OutputSignals=FR speed,RR speed,RL speed,FL speed
  Constant : Constant  Value=0
  Delay{,1..3} (4 alike) : Delay  DelayLength=1
  MC{1..4} (4 alike) : Switch  Criteria=u2 > Threshold
  Min{,1..3} (4 alike) : MinMax  Inputs=2
  MC1_trq : Outport  VectorParamsAs1DForOutWhenUnconnected=off
  MC1_targetspeed : Outport  Port=2  VectorParamsAs1DForOutWhenUnconnected=off
  CAN from INV1 : Outport  Port=3  VectorParamsAs1DForOutWhenUnconnected=off
  MC2_trq : Outport  Port=4  VectorParamsAs1DForOutWhenUnconnected=off
  MC2_targetspeed : Outport  Port=5  VectorParamsAs1DForOutWhenUnconnected=off
  CAN from INV2 : Outport  Port=6  VectorParamsAs1DForOutWhenUnconnected=off
  MC3_trq : Outport  Port=7  VectorParamsAs1DForOutWhenUnconnected=off
  MC3_targetspeed : Outport  Port=8  VectorParamsAs1DForOutWhenUnconnected=off
  CAN from INV3 : Outport  Port=9  VectorParamsAs1DForOutWhenUnconnected=off
  MC4_trq : Outport  Port=10  VectorParamsAs1DForOutWhenUnconnected=off
  MC4_targetspeed : Outport  Port=11  VectorParamsAs1DForOutWhenUnconnected=off
  CAN from INV4 : Outport  Port=12  VectorParamsAs1DForOutWhenUnconnected=off
  tag scope: FL_Torque=global, FR_Torque=global, RL_Torque=global, RR_Torque=global
  wires:
  Delay3/1 -> [FL_Torque]
  Delay2/1 -> [RL_Torque]
  Delay1/1 -> [RR_Torque]
  Delay/1 -> [FR_Torque]
  Bus Selector3/4 -> Min3/1  "<FL speed>"
  Bus Selector3/3 -> Min2/1  "<RL speed>"
  Bus Selector3/2 -> Min1/1  "<RR speed>"
  Bus Selector3/1 -> Min/1  "<FR speed>"
  Bus Selector/4 -> Delay3/1, MC4/1  "<FL trq>"
  Bus Selector/3 -> MC3/1, Delay2/1  "<RL trq>"
  Bus Selector/2 -> MC2/1, Delay1/1  "<RR trq>"
  Bus Selector/1 -> MC1/1, Delay/1  "<FR trq>"
  CAN from INV/1 -> CAN from INV1/1, CAN from INV2/1, CAN from INV3/1, CAN from INV4/1
  [speedlimit] -> Min3/2, Min2/2, Min/2, Min1/2
  TargetSpeed/1 -> Bus Selector3/1
  Min2/1 -> MC3_targetspeed/1
  Min1/1 -> MC2_targetspeed/1
  Inv select/1 -> Bus Selector2/1
  Min/1 -> MC1_targetspeed/1
  Min3/1 -> MC4_targetspeed/1
  trq Ins/1 -> Bus Selector/1
  Bus Selector2/4 -> MC4/2  "<MC4_sw>"
  Bus Selector2/3 -> MC3/2  "<MC3_sw>"
  Bus Selector2/1 -> MC1/2  "<MC1_sw>"
  Bus Selector2/2 -> MC2/2  "<MC2_sw>"
  MC3/1 -> MC3_trq/1
  MC2/1 -> MC2_trq/1
  MC1/1 -> MC1_trq/1
  MC4/1 -> MC4_trq/1
  Constant/1 -> MC4/3, MC1/3, MC2/3, MC3/3

== system VCM_main_Acc2/All Inv enable/All Inv enable ==
  CAN from Inv : Inport
  Inv select : Inport  Port=2
  All Inverter Enable : Logic  Inputs=4  AllPortsSameDT=off  OutDataTypeStr=boolean
  Bus Selector : BusSelector  OutputSignals=MC1_sw,MC2_sw,MC3_sw,MC4_sw
  Bus Selector1 : BusSelector  OutputSignals=MC_11.MC1_bQuitInverterOn,MC_21.MC2_bQuitInverterOn,MC_31.MC3_bQuitInverterOn,MC_41.MC4_bQuitInverterOn
  Constant : Constant
  Switch{1..4} (4 alike) : Switch  Criteria=u2 > Threshold
  Out1 : Outport  VectorParamsAs1DForOutWhenUnconnected=off
  wires:
  Inv select/1 -> Bus Selector/1
  CAN from Inv/1 -> Bus Selector1/1
  Switch4/1 -> All Inverter Enable/4
  Switch3/1 -> All Inverter Enable/3
  Switch1/1 -> All Inverter Enable/1
  All Inverter Enable/1 -> Out1/1
  Switch2/1 -> All Inverter Enable/2
  Constant/1 -> Switch2/3, Switch1/3, Switch3/3, Switch4/3
  Bus Selector/2 -> Switch2/2  "<MC2_sw>"
  Bus Selector/1 -> Switch1/2  "<MC1_sw>"
  Bus Selector1/3 -> Switch3/1  "<MC3_bQuitInverterOn>"
  Bus Selector1/1 -> Switch1/1  "<MC1_bQuitInverterOn>"
  Bus Selector/4 -> Switch4/2  "<MC4_sw>"
  Bus Selector/3 -> Switch3/2  "<MC3_sw>"
  Bus Selector1/2 -> Switch2/1  "<MC2_bQuitInverterOn>"
  Bus Selector1/4 -> Switch4/1  "<MC4_bQuitInverterOn>"

== system VCM_main_Acc2/Error display Box/Error Info ==
  In1 : Inport
  Bus Creator{,1..3} (4 alike) : BusCreator  Inputs=3
  Bus Creator4 : BusCreator  Inputs=4
  Bus Creator5 : BusCreator  Inputs=4
  Bus Selector : BusSelector  OutputSignals=MC_12.MC1_Diagnostic number,MC_22.MC2_Diagnostic number,MC_32.MC3_Diagnostic number,MC_42.MC4_Diagnostic number
  error memory MC1 : Subsystem
  error memory MC2 : Subsystem
  error memory MC3 : Subsystem
  error memory MC4 : Subsystem
  Out1 : Outport  VectorParamsAs1DForOutWhenUnconnected=off
  Out2 : Outport  Port=2  VectorParamsAs1DForOutWhenUnconnected=off
  wires:
  Bus Creator5/1 -> Out2/1
  Bus Creator3/1 -> Bus Creator4/4  "MC4 Error Diag"
  error memory MC4/3(error3) -> Bus Creator3/3  "Error Diag3"
  error memory MC4/4(error triger) -> Bus Creator5/4  "Error triger MC4"
  error memory MC4/2(error2) -> Bus Creator3/2  "Error Diag2"
  error memory MC4/1(error1) -> Bus Creator3/1  "Error Diag1"
  Bus Selector/4 -> error memory MC4/1(Error info)  "<MC4_Diagnostic number>"
  Bus Creator2/1 -> Bus Creator4/3  "MC3 Error Diag"
  error memory MC3/3(error3) -> Bus Creator2/3  "Error Diag3"
  error memory MC3/4(error triger) -> Bus Creator5/3  "Error triger MC3"
  error memory MC3/2(error2) -> Bus Creator2/2  "Error Diag2"
  error memory MC3/1(error1) -> Bus Creator2/1  "Error Diag1"
  Bus Selector/3 -> error memory MC3/1(Error info)  "<MC3_Diagnostic number>"
  error memory MC2/3(error3) -> Bus Creator1/3  "Error Diag3"
  error memory MC2/4(error triger) -> Bus Creator5/2  "Error triger MC2"
  Bus Creator1/1 -> Bus Creator4/2  "MC2 Error Diag"
  error memory MC2/2(error2) -> Bus Creator1/2  "Error Diag2"
  error memory MC2/1(error1) -> Bus Creator1/1  "Error Diag1"
  Bus Selector/2 -> error memory MC2/1(Error info)  "<MC2_Diagnostic number>"
  error memory MC1/3(error3) -> Bus Creator/3  "Error Diag3"
  error memory MC1/4(error triger) -> Bus Creator5/1  "Error triger MC1"
  Bus Creator4/1 -> Out1/1
  Bus Creator/1 -> Bus Creator4/1  "MC1 Error Diag"
  error memory MC1/2(error2) -> Bus Creator/2  "Error Diag2"
  error memory MC1/1(error1) -> Bus Creator/1  "Error Diag1"
  Bus Selector/1 -> error memory MC1/1(Error info)  "<MC1_Diagnostic number>"
  In1/1 -> Bus Selector/1

== system VCM_main_Acc2/Error display Box/Error Info1 ==
  In1 : Inport
  In2 : Inport  Port=2
  Bus Creator{,1..3} (4 alike) : BusCreator  Inputs=3
  Bus Creator4 : BusCreator  Inputs=4
  Bus Selector : BusSelector  OutputSignals=MC_13.MC1_Error info 1,MC_23.MC2_Error info 1,MC_33.MC3_Error info 1,MC_43.MC4_Error info 1
  Bus Selector1 : BusSelector  OutputSignals=Error triger MC1,Error triger MC2,Error triger MC3,Error triger MC4
  error memory MC1 : Subsystem
  error memory MC2 : Subsystem
  error memory MC3 : Subsystem
  error memory MC4 : Subsystem
  Out1 : Outport  VectorParamsAs1DForOutWhenUnconnected=off
  wires:
  Bus Selector/1 -> error memory MC1/1(Error info)  "<MC1_Error info 1>"
  Bus Selector1/4 -> error memory MC4/2(Error triger)  "<Error triger MC4>"
  Bus Selector1/3 -> error memory MC3/2(Error triger)  "<Error triger MC3>"
  Bus Selector1/2 -> error memory MC2/2(Error triger)  "<Error triger MC2>"
  Bus Selector1/1 -> error memory MC1/2(Error triger)  "<Error triger MC1>"
  In2/1 -> Bus Selector1/1
  Bus Selector/4 -> error memory MC4/1(Error info)  "<MC4_Error info 1>"
  Bus Selector/3 -> error memory MC3/1(Error info)  "<MC3_Error info 1>"
  Bus Selector/2 -> error memory MC2/1(Error info)  "<MC2_Error info 1>"
  error memory MC4/3(error3) -> Bus Creator3/3  "Error Diag3"
  Bus Creator3/1 -> Bus Creator4/4  "MC4 Error Diag"
  error memory MC4/2(error2) -> Bus Creator3/2  "Error Diag2"
  error memory MC4/1(error1) -> Bus Creator3/1  "Error Diag1"
  error memory MC3/3(error3) -> Bus Creator2/3  "Error Diag3"
  Bus Creator2/1 -> Bus Creator4/3  "MC3 Error Diag"
  error memory MC3/2(error2) -> Bus Creator2/2  "Error Diag2"
  error memory MC3/1(error1) -> Bus Creator2/1  "Error Diag1"
  error memory MC2/3(error3) -> Bus Creator1/3  "Error Diag3"
  Bus Creator1/1 -> Bus Creator4/2  "MC2 Error Diag"
  error memory MC2/2(error2) -> Bus Creator1/2  "Error Diag2"
  error memory MC2/1(error1) -> Bus Creator1/1  "Error Diag1"
  error memory MC1/3(error3) -> Bus Creator/3  "Error Diag3"
  Bus Creator4/1 -> Out1/1
  Bus Creator/1 -> Bus Creator4/1  "MC1 Error Diag"
  error memory MC1/2(error2) -> Bus Creator/2  "Error Diag2"
  error memory MC1/1(error1) -> Bus Creator/1  "Error Diag1"
  In1/1 -> Bus Selector/1

== system VCM_main_Acc2/Error display Box/Error Info2 ==
  In1 : Inport
  In2 : Inport  Port=2
  Bus Creator{,1..3} (4 alike) : BusCreator  Inputs=3
  Bus Creator4 : BusCreator  Inputs=4
  Bus Selector : BusSelector  OutputSignals=MC_13.MC1_Error info 1,MC_23.MC2_Error info 1,MC_33.MC3_Error info 1,MC_43.MC4_Error info 1
  Bus Selector1 : BusSelector  OutputSignals=Error triger MC1,Error triger MC2,Error triger MC3,Error triger MC4
  error memory MC1 : Subsystem
  error memory MC2 : Subsystem
  error memory MC3 : Subsystem
  error memory MC4 : Subsystem
  Out1 : Outport  VectorParamsAs1DForOutWhenUnconnected=off
  wires:
  Bus Selector1/4 -> error memory MC4/2(Error triger)  "<Error triger MC4>"
  Bus Selector1/3 -> error memory MC3/2(Error triger)  "<Error triger MC3>"
  Bus Selector1/2 -> error memory MC2/2(Error triger)  "<Error triger MC2>"
  Bus Selector1/1 -> error memory MC1/2(Error triger)  "<Error triger MC1>"
  In2/1 -> Bus Selector1/1
  Bus Selector/4 -> error memory MC4/1(Error info)  "<MC4_Error info 1>"
  Bus Selector/3 -> error memory MC3/1(Error info)  "<MC3_Error info 1>"
  Bus Selector/2 -> error memory MC2/1(Error info)  "<MC2_Error info 1>"
  error memory MC4/3(error3) -> Bus Creator3/3  "Error Diag3"
  Bus Creator3/1 -> Bus Creator4/4  "MC4 Error Diag"
  error memory MC4/2(error2) -> Bus Creator3/2  "Error Diag2"
  error memory MC4/1(error1) -> Bus Creator3/1  "Error Diag1"
  error memory MC3/3(error3) -> Bus Creator2/3  "Error Diag3"
  Bus Creator2/1 -> Bus Creator4/3  "MC3 Error Diag"
  error memory MC3/2(error2) -> Bus Creator2/2  "Error Diag2"
  error memory MC3/1(error1) -> Bus Creator2/1  "Error Diag1"
  error memory MC2/3(error3) -> Bus Creator1/3  "Error Diag3"
  Bus Creator1/1 -> Bus Creator4/2  "MC2 Error Diag"
  error memory MC2/2(error2) -> Bus Creator1/2  "Error Diag2"
  error memory MC2/1(error1) -> Bus Creator1/1  "Error Diag1"
  Bus Selector/1 -> error memory MC1/1(Error info)  "<MC1_Error info 1>"
  error memory MC1/3(error3) -> Bus Creator/3  "Error Diag3"
  Bus Creator4/1 -> Out1/1
  Bus Creator/1 -> Bus Creator4/1  "MC1 Error Diag"
  error memory MC1/2(error2) -> Bus Creator/2  "Error Diag2"
  error memory MC1/1(error1) -> Bus Creator/1  "Error Diag1"
  In1/1 -> Bus Selector/1

== system VCM_main_Acc2/Error display Box/Error Info3 ==
  In1 : Inport
  In2 : Inport  Port=2
  Bus Creator{,1..3} (4 alike) : BusCreator  Inputs=3
  Bus Creator4 : BusCreator  Inputs=4
  Bus Selector : BusSelector  OutputSignals=MC_13.MC1_Error info 1,MC_23.MC2_Error info 1,MC_33.MC3_Error info 1,MC_43.MC4_Error info 1
  Bus Selector1 : BusSelector  OutputSignals=Error triger MC1,Error triger MC2,Error triger MC3,Error triger MC4
  error memory MC1 : Subsystem
  error memory MC2 : Subsystem
  error memory MC3 : Subsystem
  error memory MC4 : Subsystem
  Out1 : Outport  VectorParamsAs1DForOutWhenUnconnected=off
  wires:
  Bus Selector/1 -> error memory MC1/1(Error info)  "<MC1_Error info 1>"
  Bus Selector1/4 -> error memory MC4/2(Error triger)  "<Error triger MC4>"
  Bus Selector1/3 -> error memory MC3/2(Error triger)  "<Error triger MC3>"
  Bus Selector1/2 -> error memory MC2/2(Error triger)  "<Error triger MC2>"
  Bus Selector1/1 -> error memory MC1/2(Error triger)  "<Error triger MC1>"
  In2/1 -> Bus Selector1/1
  Bus Selector/4 -> error memory MC4/1(Error info)  "<MC4_Error info 1>"
  Bus Selector/3 -> error memory MC3/1(Error info)  "<MC3_Error info 1>"
  Bus Selector/2 -> error memory MC2/1(Error info)  "<MC2_Error info 1>"
  error memory MC4/3(error3) -> Bus Creator3/3  "Error Diag3"
  Bus Creator3/1 -> Bus Creator4/4  "MC4 Error Diag"
  error memory MC4/2(error2) -> Bus Creator3/2  "Error Diag2"
  error memory MC4/1(error1) -> Bus Creator3/1  "Error Diag1"
  error memory MC3/3(error3) -> Bus Creator2/3  "Error Diag3"
  Bus Creator2/1 -> Bus Creator4/3  "MC3 Error Diag"
  error memory MC3/2(error2) -> Bus Creator2/2  "Error Diag2"
  error memory MC3/1(error1) -> Bus Creator2/1  "Error Diag1"
  error memory MC2/3(error3) -> Bus Creator1/3  "Error Diag3"
  Bus Creator1/1 -> Bus Creator4/2  "MC2 Error Diag"
  error memory MC2/2(error2) -> Bus Creator1/2  "Error Diag2"
  error memory MC2/1(error1) -> Bus Creator1/1  "Error Diag1"
  error memory MC1/3(error3) -> Bus Creator/3  "Error Diag3"
  Bus Creator4/1 -> Out1/1
  Bus Creator/1 -> Bus Creator4/1  "MC1 Error Diag"
  error memory MC1/2(error2) -> Bus Creator/2  "Error Diag2"
  error memory MC1/1(error1) -> Bus Creator/1  "Error Diag1"
  In1/1 -> Bus Selector/1

== system VCM_main_Acc2/Sequence/bError_SwBox ==
  BUS : Inport
  error sig1 : Inport  Port=2
  error sig2 : Inport  Port=3
  error sig3 : Inport  Port=4
  error sig4 : Inport  Port=5
  Bus Selector2 : BusSelector  OutputSignals=MC1_sw,MC2_sw,MC3_sw,MC4_sw
  Constant : Constant  Value=0
  Switch{1..4} (4 alike) : Switch  Criteria=u2 > Threshold
  Out1 : Outport  VectorParamsAs1DForOutWhenUnconnected=off
  Out2 : Outport  Port=2  VectorParamsAs1DForOutWhenUnconnected=off
  Out3 : Outport  Port=3  VectorParamsAs1DForOutWhenUnconnected=off
  Out4 : Outport  Port=4  VectorParamsAs1DForOutWhenUnconnected=off
  wires:
  error sig2/1 -> Switch2/1
  error sig3/1 -> Switch3/1
  error sig4/1 -> Switch4/1
  BUS/1 -> Bus Selector2/1
  Bus Selector2/4 -> Switch4/2  "<MC4_sw>"
  Bus Selector2/3 -> Switch3/2  "<MC3_sw>"
  Bus Selector2/1 -> Switch1/2  "<MC1_sw>"
  Bus Selector2/2 -> Switch2/2  "<MC2_sw>"
  Switch3/1 -> Out3/1
  Switch2/1 -> Out2/1
  error sig1/1 -> Switch1/1
  Switch1/1 -> Out1/1
  Switch4/1 -> Out4/1
  Constant/1 -> Switch1/3, Switch2/3, Switch3/3, Switch4/3

== system VCM_main_Acc2/Sequence/bInberterOn_SwBox1 ==
  BUS : Inport
  error sig1 : Inport  Port=2
  error sig2 : Inport  Port=3
  error sig3 : Inport  Port=4
  error sig4 : Inport  Port=5
  Bus Selector2 : BusSelector  OutputSignals=MC1_sw,MC2_sw,MC3_sw,MC4_sw
  Constant : Constant
  Switch{1..4} (4 alike) : Switch  Criteria=u2 > Threshold
  Out1 : Outport  VectorParamsAs1DForOutWhenUnconnected=off
  Out2 : Outport  Port=2  VectorParamsAs1DForOutWhenUnconnected=off
  Out3 : Outport  Port=3  VectorParamsAs1DForOutWhenUnconnected=off
  Out4 : Outport  Port=4  VectorParamsAs1DForOutWhenUnconnected=off
  wires:
  error sig2/1 -> Switch2/1
  error sig3/1 -> Switch3/1
  error sig4/1 -> Switch4/1
  BUS/1 -> Bus Selector2/1
  Bus Selector2/4 -> Switch4/2  "<MC4_sw>"
  Bus Selector2/3 -> Switch3/2  "<MC3_sw>"
  Bus Selector2/1 -> Switch1/2  "<MC1_sw>"
  Bus Selector2/2 -> Switch2/2  "<MC2_sw>"
  Switch3/1 -> Out3/1
  Switch2/1 -> Out2/1
  error sig1/1 -> Switch1/1
  Switch1/1 -> Out1/1
  Switch4/1 -> Out4/1
  Constant/1 -> Switch1/3, Switch2/3, Switch3/3, Switch4/3

== system VCM_main_Acc2/Sequence/bQuitDcOn_SwBox ==
  BUS : Inport
  error sig1 : Inport  Port=2
  error sig2 : Inport  Port=3
  error sig3 : Inport  Port=4
  error sig4 : Inport  Port=5
  Bus Selector2 : BusSelector  OutputSignals=MC1_sw,MC2_sw,MC3_sw,MC4_sw
  Constant : Constant
  Switch{1..4} (4 alike) : Switch  Criteria=u2 > Threshold
  Out1 : Outport  VectorParamsAs1DForOutWhenUnconnected=off
  Out2 : Outport  Port=2  VectorParamsAs1DForOutWhenUnconnected=off
  Out3 : Outport  Port=3  VectorParamsAs1DForOutWhenUnconnected=off
  Out4 : Outport  Port=4  VectorParamsAs1DForOutWhenUnconnected=off
  wires:
  error sig2/1 -> Switch2/1
  error sig3/1 -> Switch3/1
  error sig4/1 -> Switch4/1
  BUS/1 -> Bus Selector2/1
  Bus Selector2/4 -> Switch4/2  "<MC4_sw>"
  Bus Selector2/3 -> Switch3/2  "<MC3_sw>"
  Bus Selector2/1 -> Switch1/2  "<MC1_sw>"
  Bus Selector2/2 -> Switch2/2  "<MC2_sw>"
  Switch3/1 -> Out3/1
  Switch2/1 -> Out2/1
  error sig1/1 -> Switch1/1
  Switch1/1 -> Out1/1
  Switch4/1 -> Out4/1
  Constant/1 -> Switch1/3, Switch2/3, Switch3/3, Switch4/3

== system VCM_main_Acc2/Sequence/bSystemReady_SwBox ==
  BUS : Inport
  error sig1 : Inport  Port=2
  error sig2 : Inport  Port=3
  error sig3 : Inport  Port=4
  error sig4 : Inport  Port=5
  Bus Selector2 : BusSelector  OutputSignals=MC1_sw,MC2_sw,MC3_sw,MC4_sw
  Constant : Constant
  Switch{1..4} (4 alike) : Switch  Criteria=u2 > Threshold
  Out1 : Outport  VectorParamsAs1DForOutWhenUnconnected=off
  Out2 : Outport  Port=2  VectorParamsAs1DForOutWhenUnconnected=off
  Out3 : Outport  Port=3  VectorParamsAs1DForOutWhenUnconnected=off
  Out4 : Outport  Port=4  VectorParamsAs1DForOutWhenUnconnected=off
  wires:
  error sig2/1 -> Switch2/1
  error sig3/1 -> Switch3/1
  error sig4/1 -> Switch4/1
  BUS/1 -> Bus Selector2/1
  Bus Selector2/4 -> Switch4/2  "<MC4_sw>"
  Bus Selector2/3 -> Switch3/2  "<MC3_sw>"
  Bus Selector2/1 -> Switch1/2  "<MC1_sw>"
  Bus Selector2/2 -> Switch2/2  "<MC2_sw>"
  Switch3/1 -> Out3/1
  Switch2/1 -> Out2/1
  error sig1/1 -> Switch1/1
  Switch1/1 -> Out1/1
  Switch4/1 -> Out4/1
  Constant/1 -> Switch1/3, Switch2/3, Switch3/3, Switch4/3
